simulink model "P3_Modelo_4_2_SenalPWM"  (R2023a)
settings: Solver=VariableStepAuto  StartTime=0.0  StopTime=10.0  RelTol=1e-3
undefined symbols (not defined in the file): K
libraries: simulink x1
settings Model: Creator=sisdin  LastModifiedBy=sisdin

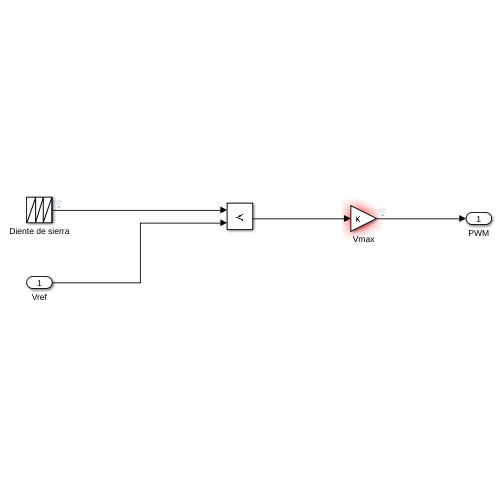
[thumbnail: Simulink's stored preview of the top-level diagram]
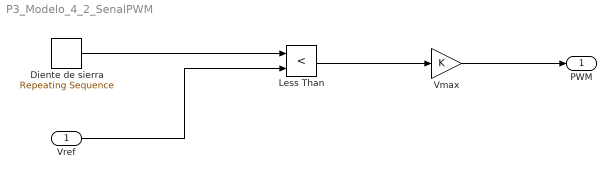
== system P3_Modelo_4_2_SenalPWM ==
  Vref : Inport
  Diente de sierra : simulink/Sources/Repeating Sequence  rep_seq_t=[0 2]  rep_seq_y=[0 2]
  Less Than : RelationalOperator  Operator=<  OutDataTypeStr=boolean  RndMeth=Simplest  InputSameDT=off
  Vmax : Gain  Gain=K
  PWM : Outport
  wires:
  Less Than/1 -> Vmax/1
  Vmax/1 -> PWM/1
  Diente de sierra/1 -> Less Than/1
  Vref/1 -> Less Than/2
